simulink library "FlagLibrary"  (R2018b)
settings: Solver=VariableStepAuto  StartTime=0.0  StopTime=10.0  RelTol=1e-3
settings Model: Creator=billg  LastModifiedBy=billg

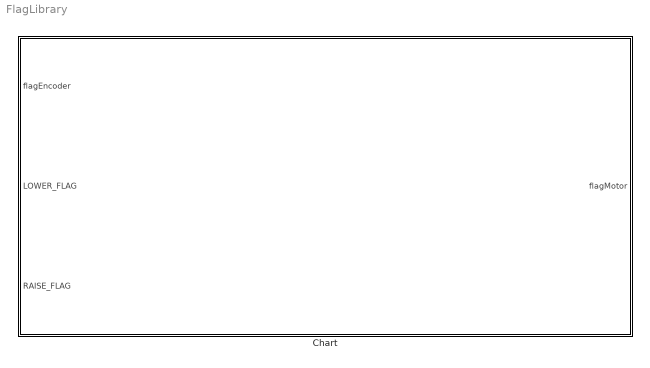
== system FlagLibrary ==
  Chart : Stateflow chart  TreatAsAtomicUnit=on

== stateflow chart FlagLibrary/Chart ==
  state Init
    entry:
    flagMotor = 0;
  state Raising
    entry:
    flagMotor = 20;
  state StartLowering
    entry:
    flagMotor = -20;
  state StopRaising
    entry:
    flagMotor = 0;
  (default) -> Init
  Init -> Raising : [RAISE_FLAG]
  StartLowering -> Init : [flagEncoder <= 0]
  Raising -> StopRaising : [flagEncoder >= 90]
  StopRaising -> StartLowering : [LOWER_FLAG]
  data: flagMotor output; flagEncoder input; LOWER_FLAG input; RAISE_FLAG input
